simulink model "test_com_SensorFusion_SF_D4_ukf"  (R2019b)
settings: Solver=FixedStepDiscrete  StartTime=0  StopTime=stop  FixedStep=0.001  RelTol=1e-3
undefined symbols (not defined in the file or in its folder): breakpoints_camber_posZ, breakpoints_camber_RollAngle, BxTM, ByTM, camber_posZ_rear, camber_RollAngle_front, camber_RollAngle_rear, CxTM, CyTM, enable_kalman_standing, enable_simpleTireLoad_pGL, enable_v2o_direct, g, gamma_stat_front, gamma_stat_rear, gearbox_ratio, l_F, l_R, m_sprung, m_unsprung_quarter, mag_calib_front_center, mag_calib_front_compmatrix, mag_calib_rear_center, mag_calib_rear_compmatrix, should_be_in_theSensorFusion, switch_lat_accel_tireloadestimE8, switch_rocker_direction_FL, switch_rocker_direction_FR, switch_rocker_direction_RL, switch_rocker_direction_RR, switch_VelYcalculation_pSF, testStart_VelX_pSF, testVelY_pSF, tire_r_dyn, track_angle_front, track_width_front, track_width_rear, v2o_x, wheel_kinematics_breakpoints, wheel_kinematics_FL_data, wheel_kinematics_FR_data, wheelbase, x9DFrontX, x9DFrontY, x9DRearX, x9DRearY
libraries: SignalProcessingSensorFusionLib x30, simulink x9
(part 3 of 9)

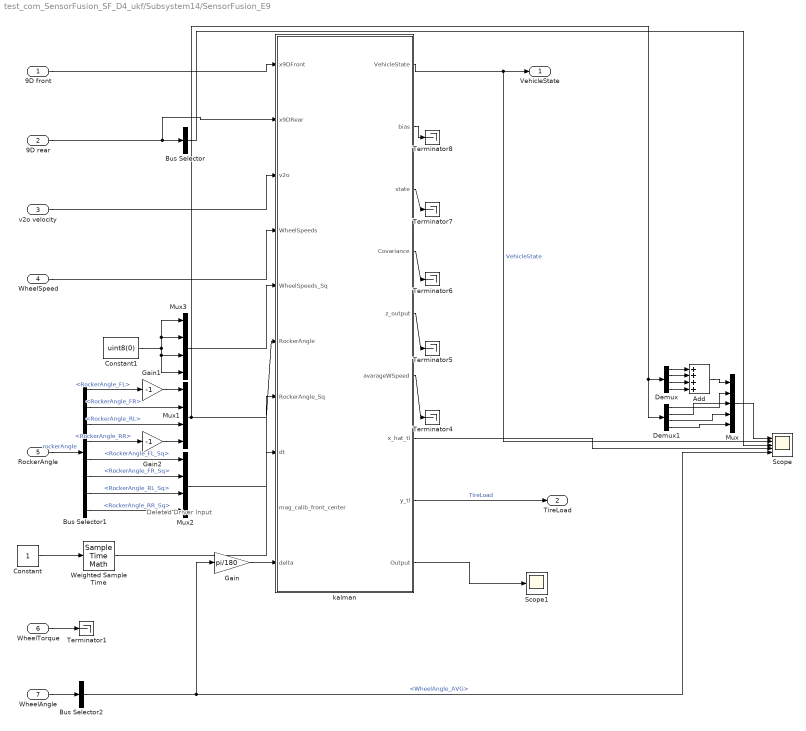
== system test_com_SensorFusion_SF_D4_ukf/Subsystem14/SensorFusion_E9 ==
  note: Deleted Driver Input
  9D front : Inport
  9D rear : Inport  Port=2
  v2o velocity : Inport  Port=3
  WheelSpeed : Inport  Port=4
  RockerAngle : Inport  Port=5
  WheelTorque : Inport  Port=6
  WheelAngle : Inport  Port=7
  Add : Sum  Inputs=++++
  Bus Selector : BusSelector  OutputSignals=AccX,AccY,AccZ,RollRate,PitchRate,YawRate  OutputAsBus=on
  Bus Selector1 : BusSelector  OutputSignals=RockerAngle_FL,RockerAngle_FR,RockerAngle_RL,RockerAngle_RR,RockerAngle_FL_Sq,RockerAngle_FR_Sq,RockerAngle_RL_Sq,RockerAngle_RR_Sq
  Bus Selector2 : BusSelector  OutputSignals=WheelAngle_AVG
  Constant : Constant
  Constant1 : Constant  Value=uint8(0)
  Demux : Demux
  Demux1 : Demux
  Gain : Gain  Gain=pi/180
  Gain1 : Gain  Gain=-1
  Gain2 : Gain  Gain=-1
  Mux : Mux  Inputs=5
  Mux1 : Mux
  Mux2 : Mux
  Mux3 : Mux
  Scope : Scope  NumInputPorts=5
  Scope1 : Scope
  Terminator{1,4..8} (6 alike) : Terminator
  Weighted Sample Time : SampleTimeMath  TsampMathOp=Ts Only
  kalman : MATLAB Function  TreatAsAtomicUnit=on
  VehicleState : Outport  VectorParamsAs1DForOutWhenUnconnected=off
  TireLoad : Outport  Port=2  VectorParamsAs1DForOutWhenUnconnected=off
  wires:
  Bus Selector1/6 -> Mux2/2  "<RockerAngle_FR_Sq>"
  kalman/1(VehicleState) -> Scope/2, VehicleState/1  "VehicleState"
  kalman/3(state) -> Terminator7/1
  Bus Selector1/2 -> Mux1/2  "<RockerAngle_FR>"
  kalman/4(Covariance) -> Terminator6/1
  Bus Selector1/1 -> Gain1/1  "<RockerAngle_FL>"
  RockerAngle/1 -> Bus Selector1/1  "rockerAngle"
  kalman/6(avarageWSpeed) -> Terminator4/1
  WheelTorque/1 -> Terminator1/1
  kalman/5(z_output) -> Terminator5/1
  Bus Selector1/4 -> Gain2/1  "<RockerAngle_RR>"
  kalman/2(bias) -> Terminator8/1
  WheelSpeed/1 -> kalman/4(WheelSpeeds)
  Bus Selector1/3 -> Mux1/3  "<RockerAngle_RL>"
  Bus Selector1/8 -> Mux2/4  "<RockerAngle_RR_Sq>"
  Bus Selector1/7 -> Mux2/3  "<RockerAngle_RL_Sq>"
  kalman/8(y_tl) -> TireLoad/1  "TireLoad"
  Constant1/1 -> Mux3/1, Mux3/2, Mux3/4, Mux3/3
  Constant/1 -> Weighted Sample Time/1
  Bus Selector1/5 -> Mux2/1  "<RockerAngle_FL_Sq>"
  WheelAngle/1 -> Bus Selector2/1
  9D rear/1 -> Bus Selector/1, kalman/2(x9DRear)
  v2o velocity/1 -> kalman/3(v2o)
  Gain1/1 -> Mux1/1
  9D front/1 -> kalman/1(x9DFront)
  Mux3/1 -> kalman/5(WheelSpeeds_Sq)
  Mux1/1 -> Demux1/1, Demux/1, kalman/6(RockerAngle)
  Mux2/1 -> kalman/7(RockerAngle_Sq)
  Weighted Sample Time/1 -> kalman/8(dt)
  Gain2/1 -> Mux1/4
  Bus Selector/1 -> Scope/3
  kalman/7(x_hat_tl) -> Scope/4
  Demux/4 -> Add/4
  Demux/3 -> Add/3
  Demux/2 -> Add/2
  Demux/1 -> Add/1
  Add/1 -> Mux/1
  Demux1/1 -> Mux/2
  Demux1/2 -> Mux/3
  Demux1/3 -> Mux/4
  Demux1/4 -> Mux/5
  Mux/1 -> Scope/1
  Bus Selector2/1 -> Scope/5, Gain/1  "<WheelAngle_AVG>"
  Gain/1 -> kalman/10(delta)
  kalman/9(Output) -> Scope1/1

== system test_com_SensorFusion_SF_D4_ukf/Subsystem14/simple_TireLoadEstimation ==
  note: Fz_FL
      | Fz_FR
      | Fz_RL
      | Fz_RR
  VehicleState : Inport  SampleTime=0.002
  Bus Selector : BusSelector  OutputSignals=AccX,AccY
  MATLAB Function : MATLAB Function  TreatAsAtomicUnit=on
  Mux2 : Mux
  TireLoad : Outport  VectorParamsAs1DForOutWhenUnconnected=off
  wires:
  Bus Selector/2 -> MATLAB Function/2(a_y)  "<AccY>"
  VehicleState/1 -> Bus Selector/1
  Bus Selector/1 -> MATLAB Function/1(a_x)  "<AccX>"
  Mux2/1 -> TireLoad/1
  MATLAB Function/1(F_z_vl) -> Mux2/1
  MATLAB Function/2(F_z_vr) -> Mux2/2
  MATLAB Function/3(F_z_hl) -> Mux2/3
  MATLAB Function/4(F_z_hr) -> Mux2/4

== system test_com_SensorFusion_SF_D4_ukf/Subsystem14/SensorFusion_D4/DriverDemand_Generation_LaunchControl ==
  DrivingMode : Inport
  PedalBrakeRecuValue : Inport  Port=2
  Pedal_BrakeMechValue : Inport  Port=3
  PedalAccelValue : Inport  Port=4
  Driver : Inport  Port=5
  Brake Map : Subsystem
  Logical Operator1 : Logic  Operator=NOT  AllPortsSameDT=off  OutDataTypeStr=boolean
  Memory : Memory  InheritSampleTime=on
  Rate Transition : RateTransition  OutPortSampleTime=0.01
  Rate Transition1 : RateTransition  OutPortSampleTime=0.01
  Saturation : Saturate  UpperLimit=0  LowerLimit=-1
  Saturation3 : Saturate  UpperLimit=1  LowerLimit=0
  Saturation4 : Saturate  UpperLimit=0  LowerLimit=-2
  Subsystem : Subsystem
  Subtract : Sum  Inputs=+-
  Switch : Switch  Criteria=u2 ~= 0
  Switch1 : Switch  Criteria=u2 > Threshold
  To Brake Torque : Gain  Gain=-1
  Totbereich Bremspedal : Subsystem
  Totbereich Gaspedal : Subsystem
  DriverDemand : Outport  VectorParamsAs1DForOutWhenUnconnected=off
  wires:
  Switch1/1 -> Switch/3  "Drive Request"
  Subtract/1 -> Saturation4/1  "Brake Request"
  To Brake Torque/1 -> Saturation/1
  Brake Map/1(DriverBrakeTorque) -> To Brake Torque/1
  Driver/1 -> Rate Transition/1
  Saturation/1 -> Subtract/1  "RecuBrake Request"
  Pedal_BrakeMechValue/1 -> Saturation3/1
  Saturation3/1 -> Subtract/2  "MechBrake Request"
  Saturation4/1 -> Switch/2, Switch/1
  Memory/1 -> Subsystem/3(DriverDemand_z), Switch1/3  "DriverDemand_z"
  DrivingMode/1 -> Rate Transition1/1
  Subsystem/1(AccelPedalEnable) -> Logical Operator1/1
  Totbereich Gaspedal/1(Drive Request) -> Subsystem/1(Drive Request), Switch1/1
  PedalAccelValue/1 -> Totbereich Gaspedal/1(Pedal_Accel_Value)
  PedalBrakeRecuValue/1 -> Totbereich Bremspedal/1(Pedal_BrakeRecu_Value)
  Totbereich Bremspedal/1(BrakeTorque) -> Brake Map/1(BrakeTorque)
  Logical Operator1/1 -> Switch1/2
  Rate Transition/1 -> Brake Map/2(Driver)
  Rate Transition1/1 -> Subsystem/2(DrivingMode)
  Switch/1 -> Memory/1, DriverDemand/1  "DriverDemand"

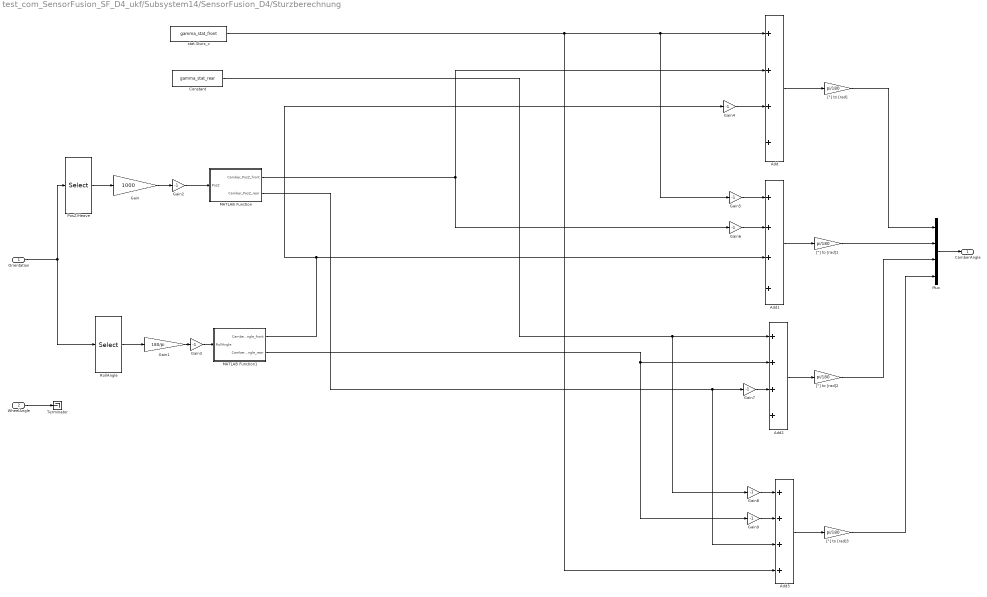
== system test_com_SensorFusion_SF_D4_ukf/Subsystem14/SensorFusion_D4/Sturzberechnung ==
  Orientation : Inport
  WheelAngle : Inport  Port=2
  Add{,1..3} (4 alike) : Sum  Inputs=++++
  Constant : Constant  Value=gamma_stat_rear
  Gain : Gain  Gain=1000  OutDataTypeStr=single
  Gain1 : Gain  Gain=180/pi
  Gain{2..9} (8 alike) : Gain  Gain=-1  OutDataTypeStr=single
  MATLAB Function : MATLAB Function  TreatAsAtomicUnit=on
  MATLAB Function1 : MATLAB Function  TreatAsAtomicUnit=on
  Mux : Mux
  PosZ/Heave : Selector  InputPortWidth=6  IndexOptions=Index vector (dialog)  Indices=1  OutputSizes=1
  RollAngle : Selector  InputPortWidth=6  IndexOptions=Index vector (dialog)  Indices=3  OutputSizes=1
  Terminator : Terminator
  "[°] to [rad]" : Gain  Gain=pi/180
  "[°] to [rad]1" : Gain  Gain=pi/180  OutDataTypeStr=single
  "[°] to [rad]2" : Gain  Gain=pi/180  OutDataTypeStr=single
  "[°] to [rad]3" : Gain  Gain=pi/180  OutDataTypeStr=single
  stat.Sturz_v : Constant  Value=gamma_stat_front
  CamberAngle : Outport  VectorParamsAs1DForOutWhenUnconnected=off
  wires:
  "[°] to [rad]"/1 -> Mux/1
  "[°] to [rad]1"/1 -> Mux/2
  "[°] to [rad]2"/1 -> Mux/3
  "[°] to [rad]3"/1 -> Mux/4
  Add/1 -> "[°] to [rad]"/1
  Add1/1 -> "[°] to [rad]1"/1
  Add2/1 -> "[°] to [rad]2"/1
  Add3/1 -> "[°] to [rad]3"/1
  stat.Sturz_v/1 -> Add3/4, Add/1, Gain5/1
  MATLAB Function/2(Camber_PosZ_rear) -> Add3/3, Gain7/1
  MATLAB Function1/2(Camber_RollAngle_rear) -> Gain9/1, Add2/2
  Orientation/1 -> RollAngle/1, PosZ/Heave/1
  Gain/1 -> Gain2/1
  PosZ/Heave/1 -> Gain/1
  RollAngle/1 -> Gain1/1
  Gain1/1 -> Gain3/1
  MATLAB Function1/1(Camber_RollAngle_front) -> Gain4/1, Add1/3
  Mux/1 -> CamberAngle/1
  WheelAngle/1 -> Terminator/1
  Gain2/1 -> MATLAB Function/1(PosZ)
  MATLAB Function/1(Camber_PosZ_front) -> Add/2, Gain6/1
  Constant/1 -> Add2/1, Gain8/1
  Gain3/1 -> MATLAB Function1/1(RollAngle)
  Gain4/1 -> Add/3
  Gain5/1 -> Add1/1
  Gain6/1 -> Add1/2
  Gain7/1 -> Add2/3
  Gain8/1 -> Add3/1
  Gain9/1 -> Add3/2

== system test_com_SensorFusion_SF_D4_ukf/Subsystem14/SensorFusion_D4/simpleTireLoadEstimation ==
  note: Fz_FL
      | Fz_FR
      | Fz_RL
      | Fz_RR
  VehicleState : Inport
  Bus Selector : BusSelector  OutputSignals=AccX,AccY
  MATLAB Function : MATLAB Function  TreatAsAtomicUnit=on
  MATLAB Function4 : MATLAB Function  TreatAsAtomicUnit=on
  Mux2 : Mux
  Scope : Scope  NumInputPorts=2
  TireLoad : Outport  VectorParamsAs1DForOutWhenUnconnected=off
  wires:
  Bus Selector/2 -> MATLAB Function/2(a_y)  "<AccY>"
  VehicleState/1 -> Bus Selector/1
  Bus Selector/1 -> Scope/1, MATLAB Function4/1(AccX)  "<AccX>"
  Mux2/1 -> TireLoad/1
  MATLAB Function/1(F_z_vl) -> Mux2/1
  MATLAB Function/2(F_z_vr) -> Mux2/2
  MATLAB Function/3(F_z_hl) -> Mux2/3
  MATLAB Function/4(F_z_hr) -> Mux2/4
  MATLAB Function4/1(AccX_out) -> Scope/2, MATLAB Function/1(a_x)

== system test_com_SensorFusion_SF_D4_ukf/Subsystem14/SensorFusion_E10/Miniaturreifenmodell Radlastdegressivität ==
  TireLoad : Inport
  NominalFricCoeff : Inport  Port=2
  Add : Sum
  Radlastdegressivität geschätzt : Lookup_n-D  NumberOfTableDimensions=1  BreakpointsForDimension1=[0:1500]  Table=-0.000001.*[0:1500].^1.8  ExtrapMethod=Clip  InternalRulePriority=Speed  RndMeth=Simplest  InputSameDT=on
  MaxFricCoeff : Outport  VectorParamsAs1DForOutWhenUnconnected=off
  wires:
  TireLoad/1 -> Radlastdegressivität geschätzt/1
  Radlastdegressivität geschätzt/1 -> Add/1  "FricCoeffLong"
  Add/1 -> MaxFricCoeff/1  "MaxFricCoeff"
  NominalFricCoeff/1 -> Add/2

== system test_com_SensorFusion_SF_D4_ukf/Subsystem14/SensorFusion_E10/Miniaturreifenmodell Radlastdegressivität1 ==
  NominalFricCoeff : Inport
  TireLoad : Inport  Port=2
  Add : Sum
  Radlastdegressivität geschätzt : Lookup_n-D  NumberOfTableDimensions=1  BreakpointsForDimension1=[0:1500]  Table=-0.000001.*[0:1500].^1.8  ExtrapMethod=Clip  InternalRulePriority=Speed  RndMeth=Simplest  InputSameDT=on
  MaxFricCoeff : Outport  VectorParamsAs1DForOutWhenUnconnected=off
  wires:
  NominalFricCoeff/1 -> Add/2
  Add/1 -> MaxFricCoeff/1  "MaxFricCoeff"
  Radlastdegressivität geschätzt/1 -> Add/1  "FricCoeffLong"
  TireLoad/1 -> Radlastdegressivität geschätzt/1

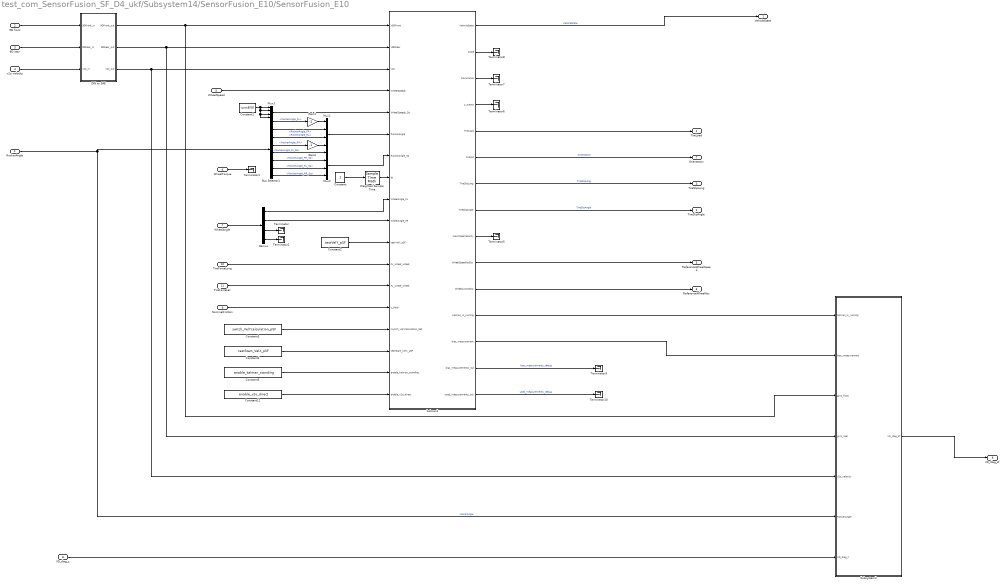
== system test_com_SensorFusion_SF_D4_ukf/Subsystem14/SensorFusion_E10/SensorFusion_E10 ==
  RockerAngle : Inport
  9D front : Inport  Port=2
  9D rear : Inport  Port=3
  v2o velocity : Inport  Port=4
  WheelSpeed : Inport  Port=5
  WheelTorque : Inport  Port=6
  WheelAngle : Inport  Port=7
  VD_diag_z : Inport  Port=8
  NominalFriction : Inport  Port=9
  TireForceLong : Inport  Port=10
  TireForceLat : Inport  Port=11
  Bus Selector1 : BusSelector  OutputSignals=RockerAngle_FL,RockerAngle_FR,RockerAngle_RL,RockerAngle_RR,RockerAngle_FL_Sq,RockerAngle_FR_Sq,RockerAngle_RL_Sq,RockerAngle_RR_Sq
  Constant : Constant
  Constant1 : Constant  Value=uint8(0)
  Constant11 : Constant  Value=enable_v2o_direct
  Constant2 : Constant  Value=testVelY_pSF  OutDataTypeStr=single
  Constant3 : Constant  Value=switch_VelYcalculation_pSF
  Constant4 : Constant  Value=testStart_VelX_pSF
  Constant5 : Constant  Value=enable_kalman_standing
  "DIN to SAE " : Subsystem
  Demux : Demux
  Gain1 : Gain  Gain=-1
  Gain2 : Gain  Gain=-1
  Mux1 : Mux
  Mux2 : Mux
  Mux3 : Mux
  Subsystem2 : Subsystem
  Terminator{,1..2,5..10} (9 alike) : Terminator
  Weighted Sample Time : SampleTimeMath  TsampMathOp=Ts Only
  kalman1 : MATLAB Function  TreatAsAtomicUnit=on
  VehicleState : Outport  VectorParamsAs1DForOutWhenUnconnected=off
  TireLoad : Outport  Port=2  VectorParamsAs1DForOutWhenUnconnected=off
  TireSlipLong : Outport  Port=3  VectorParamsAs1DForOutWhenUnconnected=off
  TireSlipAngle : Outport  Port=4  VectorParamsAs1DForOutWhenUnconnected=off
  ReferenceWheelSpeed : Outport  Port=5  VectorParamsAs1DForOutWhenUnconnected=off
  ReferenceWheelAcc : Outport  Port=6  VectorParamsAs1DForOutWhenUnconnected=off
  "Orientation " : Outport  Port=7  VectorParamsAs1DForOutWhenUnconnected=off
  VD_diag_sf : Outport  Port=8  VectorParamsAs1DForOutWhenUnconnected=off
  wires:
  Bus Selector1/6 -> Mux2/2  "<RockerAngle_FR_Sq>"
  kalman1/1(VehicleState) -> VehicleState/1  "VehicleState"
  kalman1/3(Covariance) -> Terminator7/1
  Bus Selector1/2 -> Mux1/2  "<RockerAngle_FR>"
  kalman1/4(z_output) -> Terminator6/1
  Bus Selector1/1 -> Gain1/1  "<RockerAngle_FL>"
  RockerAngle/1 -> Subsystem2/6(RockerAngle), Bus Selector1/1  "rockerAngle"
  kalman1/6(Output) -> "Orientation "/1  "Orientation"
  WheelTorque/1 -> Terminator1/1
  kalman1/9(MaxWheelVelocity) -> Terminator5/1
  Bus Selector1/4 -> Gain2/1  "<RockerAngle_RR>"
  kalman1/2(state) -> Terminator8/1
  WheelSpeed/1 -> kalman1/4(WheelSpeeds)
  Bus Selector1/3 -> Mux1/3  "<RockerAngle_RL>"
  Bus Selector1/8 -> Mux2/4  "<RockerAngle_RR_Sq>"
  Bus Selector1/7 -> Mux2/3  "<RockerAngle_RL_Sq>"
  kalman1/5(TireLoad) -> TireLoad/1
  Constant1/1 -> Mux3/2, Mux3/4, Mux3/3, Mux3/1
  Constant/1 -> Weighted Sample Time/1
  Bus Selector1/5 -> Mux2/1  "<RockerAngle_FL_Sq>"
  Gain1/1 -> Mux1/1
  Mux1/1 -> kalman1/6(RockerAngle)
  Mux2/1 -> kalman1/7(RockerAngle_Sq)
  Weighted Sample Time/1 -> kalman1/8(dt)
  Gain2/1 -> Mux1/4
  kalman1/8(TireSlipAngle) -> TireSlipAngle/1  "TireSlipAngle"
  kalman1/11(WheelAccNoSlip) -> ReferenceWheelAcc/1
  kalman1/7(TireSlipLong) -> TireSlipLong/1  "TireSlipLong"
  kalman1/10(WheelSpeedNoSlip) -> ReferenceWheelSpeed/1
  Constant2/1 -> kalman1/11(testVelY_pSF)
  TireForceLat/1 -> kalman1/13(Fy_wheel_wheel)
  TireForceLong/1 -> kalman1/12(Fx_wheel_wheel)
  NominalFriction/1 -> kalman1/14(c_Reib)
  WheelAngle/1 -> Demux/1
  Demux/3 -> Terminator/1
  Demux/4 -> Terminator2/1
  kalman1/12(kalman_is_running) -> Subsystem2/1(kalman_is_running)
  kalman1/13(bias_measurement) -> Subsystem2/2(bias_measurement)
  Demux/1 -> kalman1/9(WheelAngle_FL)
  VD_diag_z/1 -> Subsystem2/7(VD_diag_z)
  Subsystem2/1(VD_diag_sf) -> VD_diag_sf/1
  Demux/2 -> kalman1/10(WheelAngle_FR)
  Constant3/1 -> kalman1/15(switch_VelYcalculation_pSF)
  Constant4/1 -> kalman1/16(testStart_VelX_pSF)
  Constant5/1 -> kalman1/17(enable_kalman_standing)
  kalman1/15(used_measurements_out) -> Terminator10/1  "used_measurements_debug"
  kalman1/14(bias_measurements_out) -> Terminator9/1  "bias_measurements_debug"
  Constant11/1 -> kalman1/18(enable_v2o_direct)
  "DIN to SAE "/3(v2o_out) -> Subsystem2/5(v2o_velocity), kalman1/3(v2o)
  "DIN to SAE "/1(9DFront_out) -> Subsystem2/3(gyro_front), kalman1/1(x9DFront)
  "DIN to SAE "/2(9DRear_out) -> Subsystem2/4(gyro_rear), kalman1/2(x9DRear)
  9D front/1 -> "DIN to SAE "/1(9DFront_in)
  9D rear/1 -> "DIN to SAE "/2(9DRear_in)
  v2o velocity/1 -> "DIN to SAE "/3(v2o_in)
  Mux3/1 -> kalman1/5(WheelSpeeds_Sq)

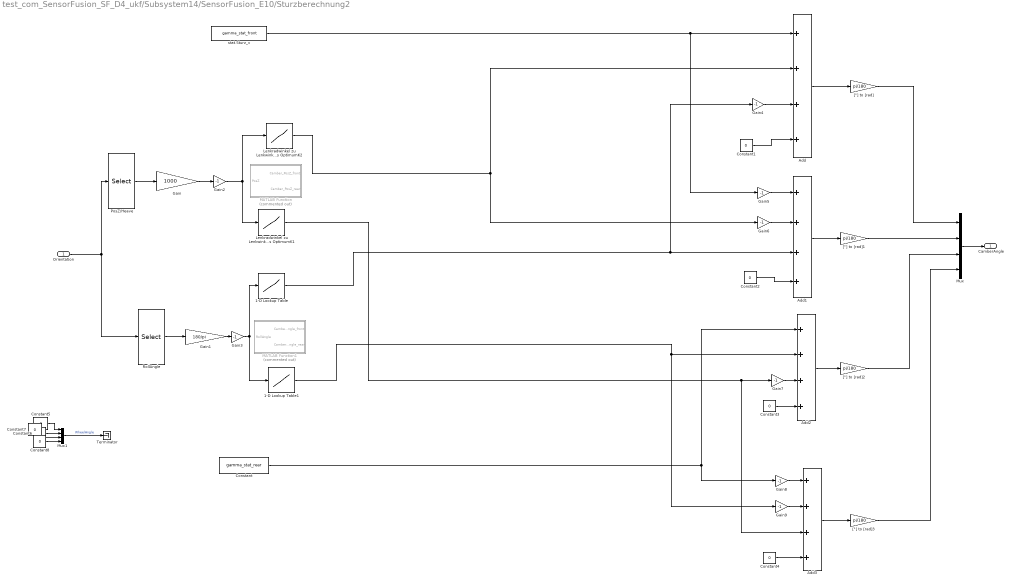
== system test_com_SensorFusion_SF_D4_ukf/Subsystem14/SensorFusion_E10/Sturzberechnung2 ==
  Orientation : Inport
  1-D Lookup Table : Lookup_n-D  NumberOfTableDimensions=1  BreakpointsForDimension1=camber_RollAngle_front  Table=breakpoints_camber_RollAngle  InternalRulePriority=Speed  RndMeth=Simplest  InputSameDT=on
  1-D Lookup Table1 : Lookup_n-D  NumberOfTableDimensions=1  BreakpointsForDimension1=camber_RollAngle_rear  Table=breakpoints_camber_RollAngle  InternalRulePriority=Speed  RndMeth=Simplest  InputSameDT=on
  Add{,1..3} (4 alike) : Sum  Inputs=++++
  Constant : Constant  Value=gamma_stat_rear  OutDataTypeStr=Inherit: Inherit via back propagation
  Constant{1..8} (8 alike) : Constant  Value=0  OutDataTypeStr=single
  Gain : Gain  Gain=1000  OutDataTypeStr=single
  Gain1 : Gain  Gain=180/pi
  Gain{2..9} (8 alike) : Gain  Gain=-1  OutDataTypeStr=single
  Lenkradwinkel zu Lenkwinkel_vl aus OptimumK1 : Lookup_n-D  NumberOfTableDimensions=1  BreakpointsForDimension1=camber_posZ_rear  Table=breakpoints_camber_posZ  InternalRulePriority=Speed  RndMeth=Simplest  InputSameDT=on
  Lenkradwinkel zu Lenkwinkel_vl aus OptimumK2 : Lookup_n-D  NumberOfTableDimensions=1  BreakpointsForDimension1=camber_posZ_rear  Table=breakpoints_camber_posZ  InternalRulePriority=Speed  RndMeth=Simplest  InputSameDT=on
  MATLAB Function : MATLAB Function  Commented=on  TreatAsAtomicUnit=on
  MATLAB Function1 : MATLAB Function  Commented=on  TreatAsAtomicUnit=on
  Mux : Mux
  Mux1 : Mux
  PosZ/Heave : Selector  InputPortWidth=6  IndexOptions=Index vector (dialog)  Indices=1  OutputSizes=1
  RollAngle : Selector  InputPortWidth=6  IndexOptions=Index vector (dialog)  Indices=3  OutputSizes=1
  Terminator : Terminator
  "[°] to [rad]" : Gain  Gain=pi/180
  "[°] to [rad]1" : Gain  Gain=pi/180  OutDataTypeStr=single
  "[°] to [rad]2" : Gain  Gain=pi/180  OutDataTypeStr=single
  "[°] to [rad]3" : Gain  Gain=pi/180  OutDataTypeStr=single
  stat.Sturz_v : Constant  Value=gamma_stat_front  OutDataTypeStr=Inherit: Inherit via back propagation
  CamberAngle : Outport  VectorParamsAs1DForOutWhenUnconnected=off
  wires:
  "[°] to [rad]"/1 -> Mux/1
  "[°] to [rad]1"/1 -> Mux/2
  "[°] to [rad]2"/1 -> Mux/3
  "[°] to [rad]3"/1 -> Mux/4
  Add/1 -> "[°] to [rad]"/1
  Add1/1 -> "[°] to [rad]1"/1
  Add2/1 -> "[°] to [rad]2"/1
  Add3/1 -> "[°] to [rad]3"/1
  Constant4/1 -> Add3/4
  Lenkradwinkel zu Lenkwinkel_vl aus OptimumK1/1 -> Add3/3, Gain7/1
  1-D Lookup Table1/1 -> Gain9/1, Add2/2
  Orientation/1 -> RollAngle/1, PosZ/Heave/1
  Gain/1 -> Gain2/1
  PosZ/Heave/1 -> Gain/1
  RollAngle/1 -> Gain1/1
  Gain1/1 -> Gain3/1
  1-D Lookup Table/1 -> Gain4/1, Add1/3
  Mux/1 -> CamberAngle/1
  Mux1/1 -> Terminator/1  "WheelAngle"
  Gain2/1 -> Lenkradwinkel zu Lenkwinkel_vl aus OptimumK2/1, Lenkradwinkel zu Lenkwinkel_vl aus OptimumK1/1
  Lenkradwinkel zu Lenkwinkel_vl aus OptimumK2/1 -> Add/2, Gain6/1
  stat.Sturz_v/1 -> Add/1, Gain5/1
  Constant/1 -> Add2/1, Gain8/1
  Gain3/1 -> 1-D Lookup Table1/1, 1-D Lookup Table/1
  Gain4/1 -> Add/3
  Gain5/1 -> Add1/1
  Gain6/1 -> Add1/2
  Gain7/1 -> Add2/3
  Gain8/1 -> Add3/1
  Gain9/1 -> Add3/2
  Constant1/1 -> Add/4
  Constant2/1 -> Add1/4
  Constant3/1 -> Add2/4
  Constant8/1 -> Mux1/4
  Constant5/1 -> Mux1/1
  Constant7/1 -> Mux1/3
  Constant6/1 -> Mux1/2

== system test_com_SensorFusion_SF_D4_ukf/Subsystem14/SensorFusion_E10/Subsystem ==
  RockerAngle : Inport
  VehicleState : Inport  Port=2
  TireLoad : Inport  Port=3
  WheelTorque : Inport  Port=4
  Constant : Constant  Value=enable_simpleTireLoad_pGL
  Constant1 : Constant  Value=[400;400;1000;1000]  OutDataTypeStr=single
  Constant2 : Constant  Value=[1000;1000;400;400]  OutDataTypeStr=single
  Multiport Switch : MultiPortSwitch  DataPortOrder=Zero-based contiguous  Inputs=4  zeroidx=on
  Sum of Elements : Sum  Inputs=+
  Terminator : Terminator
  TireLoad-Bias-Pfusch 1 : Switch  Criteria=u2 > Threshold
  TireLoadEstimationE8 : Subsystem
  simpleTireLoadEstimation : Subsystem
  TireLoad_selected : Outport  VectorParamsAs1DForOutWhenUnconnected=off
  wires:
  VehicleState/1 -> simpleTireLoadEstimation/1(VehicleState), TireLoadEstimationE8/1(VehicleState)
  TireLoadEstimationE8/2(x_hat) -> Terminator/1
  TireLoadEstimationE8/1(TireLoad) -> Multiport Switch/4  "TireLoadE8"
  TireLoad/1 -> Multiport Switch/2
  RockerAngle/1 -> TireLoadEstimationE8/2(rockerAngle)
  Constant/1 -> Multiport Switch/1
  simpleTireLoadEstimation/1(TireLoad) -> Multiport Switch/3
  Multiport Switch/1 -> TireLoad_selected/1  "TireLoad"
  WheelTorque/1 -> Sum of Elements/1
  Constant2/1 -> TireLoad-Bias-Pfusch 1/3
  Constant1/1 -> TireLoad-Bias-Pfusch 1/1
  TireLoad-Bias-Pfusch 1/1 -> Multiport Switch/5
  Sum of Elements/1 -> TireLoad-Bias-Pfusch 1/2

== system test_com_SensorFusion_SF_D4_ukf/Subsystem14/SensorFusion_E10/WheelAngle Conversion ==
  note: Anpassungen E9:
      | - Kinematikdaten für Winkelumrechnung -> mit DynamicDennis abklären
      | - TrackAngleFront als Parameter -> muss auch angepasst
  note: Annahme: Lenkrad nach links -> Negativer Lenkwinkel
      | Ausgangswinkel mathematisch positiv, von oben gesehen
  SteeringwheelAngle : Inport
  Add1 : Sum  Inputs=+-
  Add2 : Sum
  Constant : Constant  Value=0  OutDataTypeStr=single
  Constant2 : Constant  Value=0  OutDataTypeStr=single
  Data Type Conversion16 : DataTypeConversion  OutDataTypeStr=single
  Lenkradwinkel zu Lenkwinkel_vl aus OptimumK1 : Lookup_n-D  NumberOfTableDimensions=1  BreakpointsForDimension1=wheel_kinematics_breakpoints  Table=wheel_kinematics_FL_data  InternalRulePriority=Speed  RndMeth=Simplest  InputSameDT=on
  Lenkradwinkel zu Lenkwinkel_vr aus OptimumK1 : Lookup_n-D  NumberOfTableDimensions=1  BreakpointsForDimension1=wheel_kinematics_breakpoints  Table=wheel_kinematics_FR_data  InternalRulePriority=Speed  RndMeth=Simplest  InputSameDT=on
  Mux : Mux
  "[°] to [rad]" : Gain  Gain=pi/180  OutDataTypeStr=single
  "[°] to [rad]1" : Gain  Gain=pi/180  OutDataTypeStr=single
  statische_Vorspur/Nachspur_vorne : Constant  Value=track_angle_front
  WheelAngle : Outport  VectorParamsAs1DForOutWhenUnconnected=off
  wires:
  statische_Vorspur/Nachspur_vorne/1 -> Add1/2, Add2/1
  "[°] to [rad]1"/1 -> Mux/2  "WheelAngle_FR"
  Add1/1 -> "[°] to [rad]"/1  "WheelAngle_FL"
  "[°] to [rad]"/1 -> Mux/1  "WheelAngle_FL"
  Add2/1 -> "[°] to [rad]1"/1  "WheelAngle_FR"
  Lenkradwinkel zu Lenkwinkel_vl aus OptimumK1/1 -> Add1/1  "WheelAngle_FL"
  Lenkradwinkel zu Lenkwinkel_vr aus OptimumK1/1 -> Add2/2  "WheelAngle_FR"
  SteeringwheelAngle/1 -> Data Type Conversion16/1  "SteeringwheelAngle"
  Constant/1 -> Mux/3
  Constant2/1 -> Mux/4
  Mux/1 -> WheelAngle/1  "WheelAngle"
  Data Type Conversion16/1 -> Lenkradwinkel zu Lenkwinkel_vl aus OptimumK1/1, Lenkradwinkel zu Lenkwinkel_vr aus OptimumK1/1

== system test_com_SensorFusion_SF_D4_ukf/Subsystem14/SensorFusion_E10/WheelSpeed_measure ==
  In1 : Inport
  Gain19 : Gain
  Terminator19 : Terminator
  wires:
  In1/1 -> Gain19/1  "WheelSpeed"
  Gain19/1 -> Terminator19/1  "WheelSpeed_in"

== system test_com_SensorFusion_SF_D4_ukf/Subsystem14/SensorFusion_E10/simpleTireLoadEstimation ==
  note: Fz_FL
      | Fz_FR
      | Fz_RL
      | Fz_RR
  VehicleState : Inport
  Bus Selector : BusSelector  OutputSignals=AccX,AccY
  MATLAB Function : MATLAB Function  TreatAsAtomicUnit=on
  Mux2 : Mux
  TireLoad : Outport  VectorParamsAs1DForOutWhenUnconnected=off
  wires:
  Bus Selector/2 -> MATLAB Function/2(a_y)  "<AccY>"
  VehicleState/1 -> Bus Selector/1
  Bus Selector/1 -> MATLAB Function/1(a_x)  "<AccX>"
  Mux2/1 -> TireLoad/1
  MATLAB Function/1(F_z_vl) -> Mux2/1
  MATLAB Function/2(F_z_vr) -> Mux2/2
  MATLAB Function/3(F_z_hl) -> Mux2/3
  MATLAB Function/4(F_z_hr) -> Mux2/4

== system test_com_SensorFusion_SF_D4_ukf/Subsystem14/SensorFusion_E8_adjusted/SensorFusion ==
  note: DriverInput gelöscht -> bei Bedarf ChWi fragen
  9D front : Inport  SampleTime=0.002
  9D rear : Inport  Port=2  SampleTime=0.002
  v2o velocity : Inport  Port=3
  wheel speeds : Inport  Port=4
  rocker angle : Inport  Port=5
  wheel Torque : Inport  Port=6
  wheel Angle : Inport  Port=7
  Constant : Constant
  Terminator{1..4} (4 alike) : Terminator
  kalman : MATLAB Function  TreatAsAtomicUnit=on  SystemSampleTime=0.002
  VehicleState : Outport  OutDataTypeStr=Bus: control_VehicleState  VectorParamsAs1DForOutWhenUnconnected=off
  wires:
  9D rear/1 -> kalman/2(x9DRear)
  kalman/4(Covariance) -> Terminator3/1
  kalman/1(VehicleState) -> VehicleState/1
  kalman/3(Heading) -> Terminator2/1
  kalman/2(bias) -> Terminator1/1
  kalman/5(z_out) -> Terminator4/1
  9D front/1 -> kalman/1(x9DFront)
  rocker angle/1 -> kalman/5(rockerAngles)  "rockerAngle"
  Constant/1 -> kalman/8(driverInputs)
  v2o velocity/1 -> kalman/3(v2o)
  wheel speeds/1 -> kalman/4(WheelSpeeds)
  wheel Torque/1 -> kalman/6(wheelTorques)
  wheel Angle/1 -> kalman/7(wheelAngles)

== system test_com_SensorFusion_SF_D4_ukf/Subsystem14/SensorFusion_E8_adjusted/simple_TireLoadEstimation ==
  note: Fz_FL
      | Fz_FR
      | Fz_RL
      | Fz_RR
  VehicleState : Inport  SampleTime=0.002
  Bus Selector : BusSelector  OutputSignals=AccX,AccY
  MATLAB Function : MATLAB Function  TreatAsAtomicUnit=on
  Mux2 : Mux
  TireLoad : Outport  VectorParamsAs1DForOutWhenUnconnected=off
  wires:
  Bus Selector/2 -> MATLAB Function/2(a_y)  "<AccY>"
  VehicleState/1 -> Bus Selector/1
  Bus Selector/1 -> MATLAB Function/1(a_x)  "<AccX>"
  Mux2/1 -> TireLoad/1
  MATLAB Function/1(F_z_vl) -> Mux2/1
  MATLAB Function/2(F_z_vr) -> Mux2/2
  MATLAB Function/3(F_z_hl) -> Mux2/3
  MATLAB Function/4(F_z_hr) -> Mux2/4

== system test_com_SensorFusion_SF_D4_ukf/Subsystem14/SensorFusion_D4/DriverDemand_Generation_LaunchControl/Brake Map ==
  note: Bitte mit den Kennlinien unterhalb der 45 Grad Ursprungsgeraden bleiben, Einfluss auf die PowerLimitation sonst nicht auszuschließen
  note: Verschiedene Standard-Pedalmappings (ohne Geschwindigkeits- und Bremskraftfaktoreinfluss) für unterschiedliche Fahrer
  BrakeTorque : Inport
  Driver : Inport  Port=2
  AlDe : Lookup_n-D  NumberOfTableDimensions=1  BreakpointsForDimension1=[0:0.1:1]  Table=[0:0.1:1]  InternalRulePriority=Speed  RndMeth=Simplest  InputSameDT=on
  FeSch : Lookup_n-D  NumberOfTableDimensions=1  BreakpointsForDimension1=[0:0.1:1]  Table=[0:0.1:1]  InternalRulePriority=Speed  RndMeth=Simplest  InputSameDT=on
  Multiport Switch : MultiPortSwitch  DataPortOrder=Zero-based contiguous  zeroidx=on
  SiRi : Lookup_n-D  NumberOfTableDimensions=1  BreakpointsForDimension1=[0:0.1:1]  Table=[0:0.1:1]  InternalRulePriority=Speed  RndMeth=Simplest  InputSameDT=on
  DriverBrakeTorque : Outport  VectorParamsAs1DForOutWhenUnconnected=off
  wires:
  Multiport Switch/1 -> DriverBrakeTorque/1  "DriverBrakeTorque"
  BrakeTorque/1 -> AlDe/1, SiRi/1, FeSch/1
  FeSch/1 -> Multiport Switch/3
  AlDe/1 -> Multiport Switch/2
  SiRi/1 -> Multiport Switch/4
  Driver/1 -> Multiport Switch/1

== system test_com_SensorFusion_SF_D4_ukf/Subsystem14/SensorFusion_D4/DriverDemand_Generation_LaunchControl/Subsystem ==
  Drive Request : Inport
  DrivingMode : Inport  Port=2
  DriverDemand_z : Inport  Port=3
  "Aktiviere AccelPedalLogic nur in AccelModus " : simulink/Logic and Bit Operations/Compare To Constant  relop===  const=3  OutDataTypeStr=boolean
  EntryBedingung für AccelPedalLogic : simulink/Logic and Bit Operations/Compare To Constant  relop===  const=1  OutDataTypeStr=boolean
  LeaveBedingung für AccelPedalLogic : simulink/Logic and Bit Operations/Compare To Constant  relop=>=  const=0.5  OutDataTypeStr=boolean
  Logical Operator : Logic  Inputs=3  AllPortsSameDT=off  OutDataTypeStr=boolean
  AccelPedalEnable : Outport  VectorParamsAs1DForOutWhenUnconnected=off
  wires:
  EntryBedingung für AccelPedalLogic/1 -> Logical Operator/3
  LeaveBedingung für AccelPedalLogic/1 -> Logical Operator/1
  Logical Operator/1 -> AccelPedalEnable/1  "AccelPedalEnable"
  DrivingMode/1 -> "Aktiviere AccelPedalLogic nur in AccelModus "/1
  "Aktiviere AccelPedalLogic nur in AccelModus "/1 -> Logical Operator/2
  DriverDemand_z/1 -> EntryBedingung für AccelPedalLogic/1
  Drive Request/1 -> LeaveBedingung für AccelPedalLogic/1

== system test_com_SensorFusion_SF_D4_ukf/Subsystem14/SensorFusion_D4/DriverDemand_Generation_LaunchControl/Totbereich Bremspedal ==
  note: Totbereich Pedale
  Pedal_BrakeRecu_Value : Inport
  Kompensation auf ursprünglichen Wertebereich : Gain  Gain=1/0.95
  Totzone Bremspedal : DeadZone  LowerValue=0  UpperValue=0.05  SaturateOnIntegerOverflow=on
  maximaler Wert durch Totzone : Saturate  UpperLimit=0.95  LowerLimit=0
  BrakeTorque : Outport  VectorParamsAs1DForOutWhenUnconnected=off
  wires:
  maximaler Wert durch Totzone/1 -> Kompensation auf ursprünglichen Wertebereich/1
  Kompensation auf ursprünglichen Wertebereich/1 -> BrakeTorque/1  "BrakeTorque"
  Totzone Bremspedal/1 -> maximaler Wert durch Totzone/1
  Pedal_BrakeRecu_Value/1 -> Totzone Bremspedal/1  "BrakeReq"

== system test_com_SensorFusion_SF_D4_ukf/Subsystem14/SensorFusion_D4/DriverDemand_Generation_LaunchControl/Totbereich Gaspedal ==
  Pedal_Accel_Value : Inport
  Gain : Gain
  Kompensation auf ursprünglichen Wertebereich : Gain  Gain=1/0.98
  To Drive Torque : Gain
  Totzone Gaspedal : DeadZone  LowerValue=0  UpperValue=0.02  SaturateOnIntegerOverflow=on
  maximaler Wert durch Totzone : Saturate  UpperLimit=0.98  LowerLimit=0
  Drive Request : Outport  VectorParamsAs1DForOutWhenUnconnected=off
  wires:
  Totzone Gaspedal/1 -> maximaler Wert durch Totzone/1
  Gain/1 -> Totzone Gaspedal/1  "TorqueReq"
  maximaler Wert durch Totzone/1 -> Kompensation auf ursprünglichen Wertebereich/1
  To Drive Torque/1 -> Drive Request/1  "Drive Request"
  Pedal_Accel_Value/1 -> Gain/1
  Kompensation auf ursprünglichen Wertebereich/1 -> To Drive Torque/1

== system test_com_SensorFusion_SF_D4_ukf/Subsystem14/SensorFusion_E10/SensorFusion_E10/DIN to SAE  ==
  9DFront_in : Inport
  9DRear_in : Inport  Port=2
  v2o_in : Inport  Port=3
  Bus Creator : BusCreator  Inputs=7
  Bus Creator1 : BusCreator  Inputs=16
  Bus Creator2 : BusCreator  Inputs=16
  Bus Selector : BusSelector  OutputSignals=SlipAngle,VelY,VelX,SlipAngle_Sq,VelY_Sq,VelX_Sq,valueIsNew
  Bus Selector2 : BusSelector  OutputSignals=AccX,AccY,AccZ,RollRate,PitchRate,YawRate,MagX,MagY,MagZ,Temperature,AccX_Sq,AccY_Sq,AccZ_Sq,RollRate_Sq,PitchRate_Sq,YawRate_Sq
  Bus Selector3 : BusSelector  OutputSignals=AccX,AccY,AccZ,RollRate,PitchRate,YawRate,MagX,MagY,MagZ,Temperature,AccX_Sq,AccY_Sq,AccZ_Sq,RollRate_Sq,PitchRate_Sq,YawRate_Sq
  Gain{,3..12} (11 alike) : Gain  Gain=-1
  9DFront_out : Outport  VectorParamsAs1DForOutWhenUnconnected=off
  9DRear_out : Outport  Port=2  VectorParamsAs1DForOutWhenUnconnected=off
  v2o_out : Outport  Port=3  VectorParamsAs1DForOutWhenUnconnected=off
  wires:
  Bus Selector3/1 -> Bus Creator2/1  "<AccX>"
  Bus Selector3/10 -> Bus Creator2/10  "<Temperature>"
  Bus Selector2/7 -> Bus Creator1/7  "<MagX>"
  Gain3/1 -> Bus Creator1/2  "AccY"
  Bus Selector2/3 -> Gain4/1  "<AccZ>"
  Bus Selector3/8 -> Bus Creator2/8  "<MagY>"
  Bus Selector2/12 -> Bus Creator1/12  "<AccY_Sq>"
  Bus Selector2/11 -> Bus Creator1/11  "<AccX_Sq>"
  Bus Selector3/11 -> Bus Creator2/11  "<AccX_Sq>"
  Bus Creator/1 -> v2o_out/1
  Bus Creator1/1 -> 9DFront_out/1
  Bus Selector3/15 -> Bus Creator2/15  "<PitchRate_Sq>"
  Bus Selector2/2 -> Gain3/1  "<AccY>"
  Bus Selector2/4 -> Bus Creator1/4  "<RollRate>"
  Bus Selector3/5 -> Gain10/1  "<PitchRate>"
  Bus Selector2/6 -> Gain5/1  "<YawRate>"
  Bus Selector2/10 -> Bus Creator1/10  "<Temperature>"
  Bus Selector2/9 -> Gain6/1  "<MagZ>"
  Bus Selector2/5 -> Gain7/1  "<PitchRate>"
  Bus Selector3/13 -> Bus Creator2/13  "<AccZ_Sq>"
  Gain12/1 -> Bus Creator2/9  "MagZ"
  Bus Selector2/13 -> Bus Creator1/13  "<AccZ_Sq>"
  Gain9/1 -> Bus Creator2/3  "AccZ"
  Gain/1 -> Bus Creator/2  "VelY"
  Bus Selector2/8 -> Bus Creator1/8  "<MagY>"
  Gain10/1 -> Bus Creator2/5  "PitchRate"
  Bus Selector/1 -> Bus Creator/1  "<SlipAngle>"
  Bus Selector2/14 -> Bus Creator1/14  "<RollRate_Sq>"
  Bus Selector2/15 -> Bus Creator1/15  "<PitchRate_Sq>"
  Bus Creator2/1 -> 9DRear_out/1
  Bus Selector2/16 -> Bus Creator1/16  "<YawRate_Sq>"
  Bus Selector/6 -> Bus Creator/6  "<VelX_Sq>"
  Bus Selector2/1 -> Bus Creator1/1  "<AccX>"
  Gain11/1 -> Bus Creator2/6  "YawRate"
  Gain6/1 -> Bus Creator1/9  "MagZ"
  Bus Selector3/3 -> Gain9/1  "<AccZ>"
  Bus Selector3/6 -> Gain11/1  "<YawRate>"
  Bus Selector3/4 -> Bus Creator2/4  "<RollRate>"
  Bus Selector/7 -> Bus Creator/7  "<valueIsNew>"
  Bus Selector3/7 -> Bus Creator2/7  "<MagX>"
  v2o_in/1 -> Bus Selector/1
  Bus Selector3/12 -> Bus Creator2/12  "<AccY_Sq>"
  Bus Selector3/14 -> Bus Creator2/14  "<RollRate_Sq>"
  Bus Selector/5 -> Bus Creator/5  "<VelY_Sq>"
  Bus Selector3/9 -> Gain12/1  "<MagZ>"
  Bus Selector3/16 -> Bus Creator2/16  "<YawRate_Sq>"
  Bus Selector3/2 -> Gain8/1  "<AccY>"
  Bus Selector/3 -> Bus Creator/3  "<VelX>"
  Bus Selector/2 -> Gain/1  "<VelY>"
  Gain8/1 -> Bus Creator2/2  "AccY"
  Gain7/1 -> Bus Creator1/5  "PitchRate"
  Gain4/1 -> Bus Creator1/3  "AccZ"
  9DFront_in/1 -> Bus Selector2/1
  Bus Selector/4 -> Bus Creator/4  "<SlipAngle_Sq>"
  Gain5/1 -> Bus Creator1/6  "YawRate"
  9DRear_in/1 -> Bus Selector3/1

== system test_com_SensorFusion_SF_D4_ukf/Subsystem14/SensorFusion_E10/SensorFusion_E10/Subsystem2 ==
  kalman_is_running : Inport
  bias_measurement : Inport  Port=2
  gyro_front : Inport  Port=3
  gyro_rear : Inport  Port=4
  v2o_velocity : Inport  Port=5
  RockerAngle : Inport  Port=6
  VD_diag_z : Inport  Port=7
  9D_front_measure : Subsystem
  9D_rear_measure : Subsystem
  MATLAB Function1 : MATLAB Function  TreatAsAtomicUnit=on
  RT : RateTransition  OutPortSampleTime=0.002
  RockerAngle_measure : Subsystem
  Subsystem1 : Subsystem
  v2o_measure : Subsystem
  VD_diag_sf : Outport  VectorParamsAs1DForOutWhenUnconnected=off
  wires:
  9D_rear_measure/1(VD_diag_9Drear) -> MATLAB Function1/2(VD_diag_9Drear)
  gyro_rear/1 -> 9D_rear_measure/1(gyro_rear)
  gyro_front/1 -> 9D_front_measure/1(gyro_front)
  bias_measurement/1 -> Subsystem1/3(bias_measurement)
  MATLAB Function1/1(sensorFail) -> Subsystem1/4(sensorFail)
  RockerAngle/1 -> RockerAngle_measure/1(RockerAngle)
  9D_front_measure/1(VD_diag_9Dfront) -> MATLAB Function1/1(VD_diag_9Dfront)
  VD_diag_z/1 -> Subsystem1/1(VD_Diag_z)
  v2o_velocity/1 -> v2o_measure/1(v2o_velocity)
  kalman_is_running/1 -> Subsystem1/2("kalmanRunning ")
  Subsystem1/1(VD_Diag_sf) -> VD_diag_sf/1
  v2o_measure/1(VD_diag_v2o) -> RT/1
  RockerAngle_measure/1(VD_diag_RockerAngle) -> MATLAB Function1/4(VD_diag_RockerAngle)
  RT/1 -> MATLAB Function1/3(VD_diag_v2o)

== system test_com_SensorFusion_SF_D4_ukf/Subsystem14/SensorFusion_E10/Subsystem/TireLoadEstimationE8 ==
  note: z
      | z_dot
      | phi
      | phi_dot
      | theta
      | theta_dot
  note: hs_FL
      | hs_FR
      | hs_RL
      | hs_RR
  note: Fz_FL
      | Fz_FR
      | Fz_RL
      | Fz_RR
  VehicleState : Inport
  rockerAngle : Inport  Port=2
  Bus Selector : BusSelector  OutputSignals=AccX,AccY,VelX
  Bus Selector1 : BusSelector  OutputSignals=RockerAngle_FL,RockerAngle_FR,RockerAngle_RL,RockerAngle_RR
  Demux : Demux
  Demux16 : Demux  Outputs=10
  Demux17 : Demux
  Gain : Gain  Gain=-1
  Gain1 : Gain  Gain=-1
  Gain2 : Gain  Gain=switch_rocker_direction_FL
  Gain3 : Gain  Gain=switch_rocker_direction_FR
  Gain4 : Gain  Gain=switch_rocker_direction_RL
  Gain5 : Gain  Gain=switch_rocker_direction_RR
  Gain6 : Gain  Gain=switch_lat_accel_tireloadestimE8
  Mux : Mux  Inputs=3
  Mux1 : Mux
  Mux2 : Mux
  P_diag_E8 : Scope  NumInputPorts=10
  Terminator1 : Terminator
  offset_E8 : Scope  NumInputPorts=4
  "tireload estimator " : MATLAB Function  TreatAsAtomicUnit=on
  TireLoad : Outport  VectorParamsAs1DForOutWhenUnconnected=off
  x_hat : Outport  Port=2  VectorParamsAs1DForOutWhenUnconnected=off
  wires:
  Demux16/7 -> P_diag_E8/7
  rockerAngle/1 -> Bus Selector1/1
  Bus Selector1/3 -> Gain4/1  "<RockerAngle_RL>"
  "tireload estimator "/5(lp) -> Terminator1/1
  "tireload estimator "/2(y) -> Demux/1
  Bus Selector1/2 -> Gain3/1  "<RockerAngle_FR>"
  Demux16/2 -> P_diag_E8/2
  Demux17/4 -> offset_E8/4
  Demux17/2 -> offset_E8/2
  Demux17/3 -> offset_E8/3
  Bus Selector1/4 -> Gain5/1  "<RockerAngle_RR>"
  Demux16/4 -> P_diag_E8/4
  Bus Selector/2 -> Gain6/1  "<AccY>"
  Demux16/8 -> P_diag_E8/8
  Demux17/1 -> offset_E8/1
  VehicleState/1 -> Bus Selector/1
  Bus Selector1/1 -> Gain2/1  "<RockerAngle_FL>"
  Demux16/9 -> P_diag_E8/9
  Bus Selector/1 -> Mux/1  "<AccX>"
  Demux16/10 -> P_diag_E8/10
  Demux16/3 -> P_diag_E8/3
  "tireload estimator "/4(offset) -> Demux17/1
  "tireload estimator "/1(x_hat) -> x_hat/1
  Mux2/1 -> TireLoad/1
  Demux16/1 -> P_diag_E8/1
  Demux16/6 -> P_diag_E8/6
  Demux16/5 -> P_diag_E8/5
  Mux/1 -> "tireload estimator "/1(u_in)
  Gain/1 -> Mux1/1
  Gain1/1 -> Mux1/3
  Bus Selector/3 -> Mux/3  "<VelX>"
  Mux1/1 -> "tireload estimator "/2(z)
  "tireload estimator "/3(P_diag) -> Demux16/1
  Demux/1 -> Mux2/1
  Demux/2 -> Mux2/2
  Demux/3 -> Mux2/3
  Demux/4 -> Mux2/4
  Gain2/1 -> Gain/1
  Gain3/1 -> Mux1/2
  Gain4/1 -> Gain1/1
  Gain5/1 -> Mux1/4
  Gain6/1 -> Mux/2

== system test_com_SensorFusion_SF_D4_ukf/Subsystem14/SensorFusion_E10/Subsystem/simpleTireLoadEstimation ==
  note: Fz_FL
      | Fz_FR
      | Fz_RL
      | Fz_RR
  VehicleState : Inport
  Bus Selector : BusSelector  OutputSignals=AccX,AccY
  MATLAB Function : MATLAB Function  TreatAsAtomicUnit=on
  Mux2 : Mux
  TireLoad : Outport  VectorParamsAs1DForOutWhenUnconnected=off
  wires:
  Bus Selector/2 -> MATLAB Function/2(a_y)  "<AccY>"
  VehicleState/1 -> Bus Selector/1
  Bus Selector/1 -> MATLAB Function/1(a_x)  "<AccX>"
  Mux2/1 -> TireLoad/1
  MATLAB Function/1(F_z_vl) -> Mux2/1
  MATLAB Function/2(F_z_vr) -> Mux2/2
  MATLAB Function/3(F_z_hl) -> Mux2/3
  MATLAB Function/4(F_z_hr) -> Mux2/4

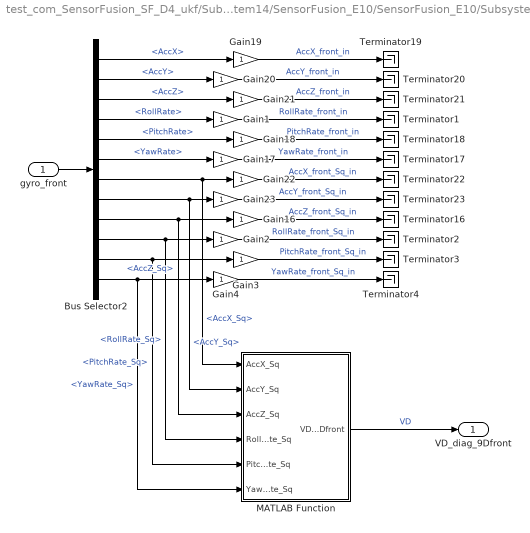
== system test_com_SensorFusion_SF_D4_ukf/Subsystem14/SensorFusion_E10/SensorFusion_E10/Subsystem2/9D_front_measure ==
  gyro_front : Inport
  Bus Selector2 : BusSelector  OutputSignals=AccX,AccY,AccZ,RollRate,PitchRate,YawRate,AccX_Sq,AccY_Sq,AccZ_Sq,RollRate_Sq,PitchRate_Sq,YawRate_Sq
  Gain{1..4,16..23} (12 alike) : Gain
  MATLAB Function : MATLAB Function  TreatAsAtomicUnit=on
  Terminator{1..4,16..23} (12 alike) : Terminator
  VD_diag_9Dfront : Outport  VectorParamsAs1DForOutWhenUnconnected=off
  wires:
  Gain22/1 -> Terminator22/1  "AccX_front_Sq_in"
  Gain21/1 -> Terminator21/1  "AccZ_front_in"
  Gain18/1 -> Terminator18/1  "PitchRate_front_in"
  Gain19/1 -> Terminator19/1  "AccX_front_in"
  Gain20/1 -> Terminator20/1  "AccY_front_in"
  Gain17/1 -> Terminator17/1  "YawRate_front_in"
  Bus Selector2/5 -> Gain18/1  "<PitchRate>"
  Gain16/1 -> Terminator16/1  "AccZ_front_Sq_in"
  Bus Selector2/3 -> Gain21/1  "<AccZ>"
  Gain23/1 -> Terminator23/1  "AccY_front_Sq_in"
  Bus Selector2/7 -> MATLAB Function/1(AccX_Sq), Gain22/1  "<AccX_Sq>"
  Bus Selector2/1 -> Gain19/1  "<AccX>"
  Bus Selector2/9 -> MATLAB Function/3(AccZ_Sq), Gain16/1  "<AccZ_Sq>"
  Bus Selector2/6 -> Gain17/1  "<YawRate>"
  Bus Selector2/8 -> MATLAB Function/2(AccY_Sq), Gain23/1  "<AccY_Sq>"
  Bus Selector2/2 -> Gain20/1  "<AccY>"
  gyro_front/1 -> Bus Selector2/1
  Gain1/1 -> Terminator1/1  "RollRate_front_in"
  Bus Selector2/4 -> Gain1/1  "<RollRate>"
  Bus Selector2/12 -> MATLAB Function/6(YawRate_Sq), Gain4/1  "<YawRate_Sq>"
  Bus Selector2/10 -> MATLAB Function/4(RollRate_Sq), Gain2/1  "<RollRate_Sq>"
  Bus Selector2/11 -> MATLAB Function/5(PitchRate_Sq), Gain3/1  "<PitchRate_Sq>"
  Gain4/1 -> Terminator4/1  "YawRate_front_Sq_in"
  Gain2/1 -> Terminator2/1  "RollRate_front_Sq_in"
  Gain3/1 -> Terminator3/1  "PitchRate_front_Sq_in"
  MATLAB Function/1(VD_diag_9Dfront) -> VD_diag_9Dfront/1  "VD"

== system test_com_SensorFusion_SF_D4_ukf/Subsystem14/SensorFusion_E10/SensorFusion_E10/Subsystem2/9D_rear_measure ==
  gyro_rear : Inport
  Bus Selector2 : BusSelector  OutputSignals=AccX,AccY,AccZ,RollRate,PitchRate,YawRate,AccX_Sq,AccY_Sq,AccZ_Sq,RollRate_Sq,PitchRate_Sq,YawRate_Sq
  Gain{1..4,16..23} (12 alike) : Gain
  MATLAB Function : MATLAB Function  TreatAsAtomicUnit=on
  Terminator{1..4,16..23} (12 alike) : Terminator
  VD_diag_9Drear : Outport  VectorParamsAs1DForOutWhenUnconnected=off
  wires:
  Gain3/1 -> Terminator3/1  "PitchRate_rear_Sq_in"
  Gain2/1 -> Terminator2/1  "RollRate_rear_Sq_in"
  Gain4/1 -> Terminator4/1  "YawRate_rear_Sq_in"
  Bus Selector2/11 -> MATLAB Function/5(PitchRate_Sq), Gain3/1  "<PitchRate_Sq>"
  Bus Selector2/10 -> MATLAB Function/4(YawRate_Sq), Gain2/1  "<RollRate_Sq>"
  Bus Selector2/12 -> MATLAB Function/6(RollRate_Sq), Gain4/1  "<YawRate_Sq>"
  Bus Selector2/4 -> Gain1/1  "<RollRate>"
  Gain1/1 -> Terminator1/1  "RollRate_rear_in"
  gyro_rear/1 -> Bus Selector2/1
  Bus Selector2/2 -> Gain20/1  "<AccY>"
  Bus Selector2/8 -> MATLAB Function/2(AccY_Sq), Gain23/1  "<AccY_Sq>"
  Bus Selector2/6 -> Gain17/1  "<YawRate>"
  Bus Selector2/9 -> MATLAB Function/3(AccZ_Sq), Gain16/1  "<AccZ_Sq>"
  Bus Selector2/1 -> Gain19/1  "<AccX>"
  Bus Selector2/7 -> MATLAB Function/1(AccX_Sq), Gain22/1  "<AccX_Sq>"
  Gain23/1 -> Terminator23/1  "AccY_rear_Sq_in"
  Bus Selector2/3 -> Gain21/1  "<AccZ>"
  Gain16/1 -> Terminator16/1  "AccZ_rear_Sq_in"
  Bus Selector2/5 -> Gain18/1  "<PitchRate>"
  Gain17/1 -> Terminator17/1  "YawRate_rear_in"
  Gain20/1 -> Terminator20/1  "AccY_rear_in"
  Gain19/1 -> Terminator19/1  "AccX_rear_in"
  Gain18/1 -> Terminator18/1  "PitchRate_rear_in"
  Gain21/1 -> Terminator21/1  "AccZ_rear_in"
  Gain22/1 -> Terminator22/1  "AccX_rear_Sq_in"
  MATLAB Function/1(VD_diag_9Drear) -> VD_diag_9Drear/1

== system test_com_SensorFusion_SF_D4_ukf/Subsystem14/SensorFusion_E10/SensorFusion_E10/Subsystem2/RockerAngle_measure ==
  RockerAngle : Inport
  Bus Selector2 : BusSelector  OutputSignals=RockerAngle_FL,RockerAngle_FR,RockerAngle_RL,RockerAngle_RR,RockerAngle_FL_Sq,RockerAngle_FR_Sq,RockerAngle_RL_Sq,RockerAngle_RR_Sq
  Gain{1,17..23} (8 alike) : Gain
  MATLAB Function : MATLAB Function  TreatAsAtomicUnit=on
  Terminator{1,17..23} (8 alike) : Terminator
  VD_diag_RockerAngle : Outport  VectorParamsAs1DForOutWhenUnconnected=off
  wires:
  Gain22/1 -> Terminator22/1  "RockerAngle_RL_Sq_in"
  Gain21/1 -> Terminator21/1  "RockerAngle_RL_in"
  Gain18/1 -> Terminator18/1  "RockerAngle_FL_Sq_in"
  Gain19/1 -> Terminator19/1  "RockerAngle_FL_in"
  Gain20/1 -> Terminator20/1  "RockerAngle_FR_in"
  Gain17/1 -> Terminator17/1  "RockerAngle_FR_Sq_in"
  Bus Selector2/5 -> Gain18/1, MATLAB Function/1(RockerAngle_FL_Sq)  "<RockerAngle_FL_Sq>"
  Bus Selector2/3 -> Gain21/1  "<RockerAngle_RL>"
  Gain23/1 -> Terminator23/1  "RockerAngle_RR_Sq_in"
  Bus Selector2/7 -> MATLAB Function/3(RockerAngle_RL_Sq), Gain22/1  "<RockerAngle_RL_Sq>"
  Bus Selector2/1 -> Gain19/1  "<RockerAngle_FL>"
  Bus Selector2/6 -> MATLAB Function/2(RockerAngle_FR_Sq), Gain17/1  "<RockerAngle_FR_Sq>"
  Bus Selector2/8 -> MATLAB Function/4(RockerAngle_RR_Sq), Gain23/1  "<RockerAngle_RR_Sq>"
  Bus Selector2/2 -> Gain20/1  "<RockerAngle_FR>"
  RockerAngle/1 -> Bus Selector2/1
  Gain1/1 -> Terminator1/1  "RockerAngle_RR_in"
  Bus Selector2/4 -> Gain1/1  "<RockerAngle_RR>"
  MATLAB Function/1(VD_diag_RockerAngle) -> VD_diag_RockerAngle/1

== system test_com_SensorFusion_SF_D4_ukf/Subsystem14/SensorFusion_E10/SensorFusion_E10/Subsystem2/Subsystem1 ==
  VD_Diag_z : Inport  OutDataTypeStr=uint32
  "kalmanRunning " : Inport  Port=2
  bias_measurement : Inport  Port=3
  sensorFail : Inport  Port=4
  Bit Clear : simulink/Logic and Bit Operations/Bit Clear  iBit=EKF_running_bit_pGL
      settings: SourceProductName=Simulink  SourceProductBaseCode=SL
  Bit Clear1 : simulink/Logic and Bit Operations/Bit Clear  iBit=Bias_measurement_running_bit_pGL
      settings: SourceProductName=Simulink  SourceProductBaseCode=SL
  Bit Clear2 : simulink/Logic and Bit Operations/Bit Clear  iBit=Sensor_Implausible_bit_pGL
      settings: SourceProductName=Simulink  SourceProductBaseCode=SL
  Bit Set : simulink/Logic and Bit Operations/Bit Set  iBit=EKF_running_bit_pGL
      settings: SourceProductName=Simulink  SourceProductBaseCode=SL
  Bit Set1 : simulink/Logic and Bit Operations/Bit Set  iBit=Bias_measurement_running_bit_pGL
      settings: SourceProductName=Simulink  SourceProductBaseCode=SL
  Bit Set2 : simulink/Logic and Bit Operations/Bit Set  iBit=Sensor_Implausible_bit_pGL
      settings: SourceProductName=Simulink  SourceProductBaseCode=SL
  RT : RateTransition  OutPortSampleTime=0.001
  Switch1 : Switch  Criteria=u2 > Threshold
  Switch2 : Switch  Criteria=u2 > Threshold
  Switch4 : Switch  Criteria=u2 > Threshold
  VD_Diag_sf : Outport  VectorParamsAs1DForOutWhenUnconnected=off
  wires:
  "kalmanRunning "/1 -> Switch4/2
  VD_Diag_z/1 -> Bit Clear/1, Bit Set/1
  Switch4/1 -> Bit Clear1/1, Bit Set1/1
  Switch1/1 -> Bit Clear2/1, Bit Set2/1
  bias_measurement/1 -> Switch1/2
  Bit Clear1/1 -> Switch1/3
  Bit Set1/1 -> Switch1/1
  Bit Clear2/1 -> Switch2/3
  Bit Set2/1 -> Switch2/1
  Switch2/1 -> VD_Diag_sf/1  "VD_Diag_sf"
  sensorFail/1 -> Switch2/2
  Bit Set/1 -> Switch4/1
  Bit Clear/1 -> RT/1
  RT/1 -> Switch4/3

== system test_com_SensorFusion_SF_D4_ukf/Subsystem14/SensorFusion_E10/SensorFusion_E10/Subsystem2/v2o_measure ==
  v2o_velocity : Inport
  Bus Selector2 : BusSelector  OutputSignals=VelY,VelX,VelY_Sq,VelX_Sq,valueIsNew
  Gain{1,18..21} (5 alike) : Gain
  MATLAB Function : MATLAB Function  TreatAsAtomicUnit=on
  Terminator{1,18..21} (5 alike) : Terminator
  VD_diag_v2o : Outport  VectorParamsAs1DForOutWhenUnconnected=off
  wires:
  Gain21/1 -> Terminator21/1  "VelY_Sq_in"
  Gain18/1 -> Terminator18/1  "valueIsNew_in"
  Gain19/1 -> Terminator19/1  "VelY_in"
  Gain20/1 -> Terminator20/1  "VelX_in"
  Bus Selector2/5 -> Gain18/1  "<valueIsNew>"
  Bus Selector2/3 -> MATLAB Function/2(VelY_Sq), Gain21/1  "<VelY_Sq>"
  Bus Selector2/1 -> Gain19/1  "<VelY>"
  Bus Selector2/2 -> Gain20/1  "<VelX>"
  v2o_velocity/1 -> Bus Selector2/1
  Gain1/1 -> Terminator1/1  "VelX_Sq_in"
  Bus Selector2/4 -> MATLAB Function/1(VelX_Sq), Gain1/1  "<VelX_Sq>"
  MATLAB Function/1(VD_diag_v2o) -> VD_diag_v2o/1
